simulink library "Lib_Turbo_Burner_TMATS_new"  (R2015a)
settings: Solver=ode45  StartTime=0.0  StopTime=10.0  RelTol=1e-3
Description:
  | Thomas Modules
settings Model: Creator=jwchapm2  LastModifiedBy=jwhitfie
settings OptimizationCC: ExpressionDepthLimit=2147483647
settings DebuggingCC: UnderspecifiedInitializationDetection=Classic  MergeDetectMultiDrivingBlocksExec=none  SolverPrmCheckMsg=warning  StateNameClashWarn=warning

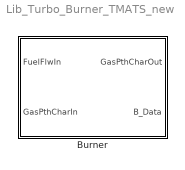
== system Lib_Turbo_Burner_TMATS_new ==
  Burner : Subsystem  mask(T-MATS: Burner Library Block){LHVEn_M=on, LHV_M=18400, Eff_M=1, hFuel_M=-1200, dPnormBurner_M=0.05}
      mask prompts: LHVEn_M "LHVEn_M - fuel LHV enabled (check use LHV method, unchecked use hFuel"; LHV_M "LHV_M - Fuel Lower Heating Value  (BTU/lb)"; Eff_M "Eff_M - Burner Efficiency [frac]"; hFuel_M "hFuel_M - Fuel enthalpy (BTU/lbm)"; dPnormBurner_M "dPnormBurner_M - Normalized Burner deltaP (1 - psi/psi)"
      mask help: This block simulates the performance of a burner using basic thermodynamic equations and properties.
      mask Help: web(which('Turbo_TMATS_Brn.html'),'-helpbrowser')
      mask Callback LHVEn_M:
      | MSK_SEC_Enables_TMATS('LHVEn_M',[2 3],'en')
      | MSK_SEC_Enables_TMATS('LHVEn_M',[4],'dis')

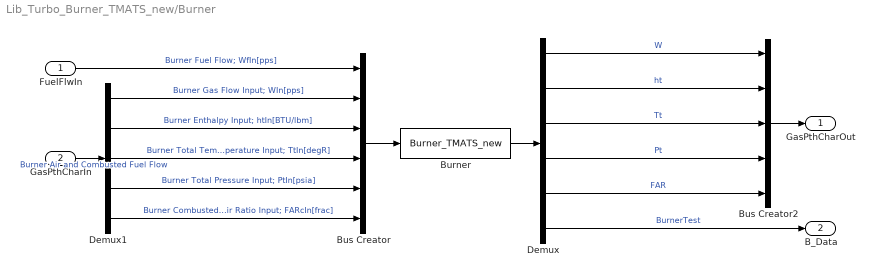
== system Lib_Turbo_Burner_TMATS_new/Burner ==
  FuelFlwIn : Inport
  GasPthCharIn : Inport  Port=2
  Burner : S-Function  FunctionName=Burner_TMATS_new  Parameters=LHV_M, dPnormBurner_M, Eff_M, LHVEn_M, hFuel_M  SFunctionModules='h2tc_TMATS t2hc_TMATS functions_TMATS'  SFunctionDeploymentMode=off  EnableBusSupport=off
  Bus Creator : BusCreator  Inputs=6
  Bus Creator2 : BusCreator  Inputs=5
  Demux : Demux  Outputs=6
  Demux1 : Demux  Outputs=5
  GasPthCharOut : Outport
  B_Data : Outport  Port=2
  wires:
  FuelFlwIn/1 -> Bus Creator/1  "Burner Fuel Flow; WfIn[pps]"
  Demux1/1 -> Bus Creator/2  "Burner Gas Flow Input; WIn[pps]"
  Burner/1 -> Demux/1
  Demux/1 -> Bus Creator2/1  "W"
  Demux/5 -> Bus Creator2/5  "FAR"
  Bus Creator/1 -> Burner/1
  Demux/6 -> B_Data/1  "BurnerTest"
  Demux1/4 -> Bus Creator/5  "Burner Total Pressure Input; PtIn[psia]"
  Demux1/3 -> Bus Creator/4  "Burner Total Temperature Input; TtIn[degR]"
  Demux1/5 -> Bus Creator/6  "Burner Combusted Fuel to Air Ratio Input; FARcIn[frac]"
  Demux/2 -> Bus Creator2/2  "ht"
  Demux/3 -> Bus Creator2/3  "Tt"
  Demux/4 -> Bus Creator2/4  "Pt"
  Bus Creator2/1 -> GasPthCharOut/1
  GasPthCharIn/1 -> Demux1/1  "Burner Air and Combusted Fuel Flow"
  Demux1/2 -> Bus Creator/3  "Burner Enthalpy Input; htIn[BTU/lbm]"
